simulink model "P3"  (R2017b)
settings: Solver=VariableStepAuto  StartTime=0.0  StopTime=10.0  RelTol=1e-3
values from neighbouring files (symbols this model uses):
  a = [0 1;-1 -0.7]    [P2a.m]    (also in P2b.m; P2c.m)
  b = [0;1]    [P2a.m]    (also in P2b.m; P2c.m)
  c = [1 0;0 0]    [P2a.m]    (also in P2b.m; P2c.m = [1 0)
  P0 = 100*eye(2)    [P2c.m]
  Q = eye(2)    [P2a.m]    (also in P2b.m; P2c.m)
  R = eye(1)    [P2a.m]    (also in P2b.m; P2c.m)
undefined symbols (not defined in the file or in its folder): H_k1, K, L
settings Model: Creator=Soutrik  LastModifiedBy=Soutrik

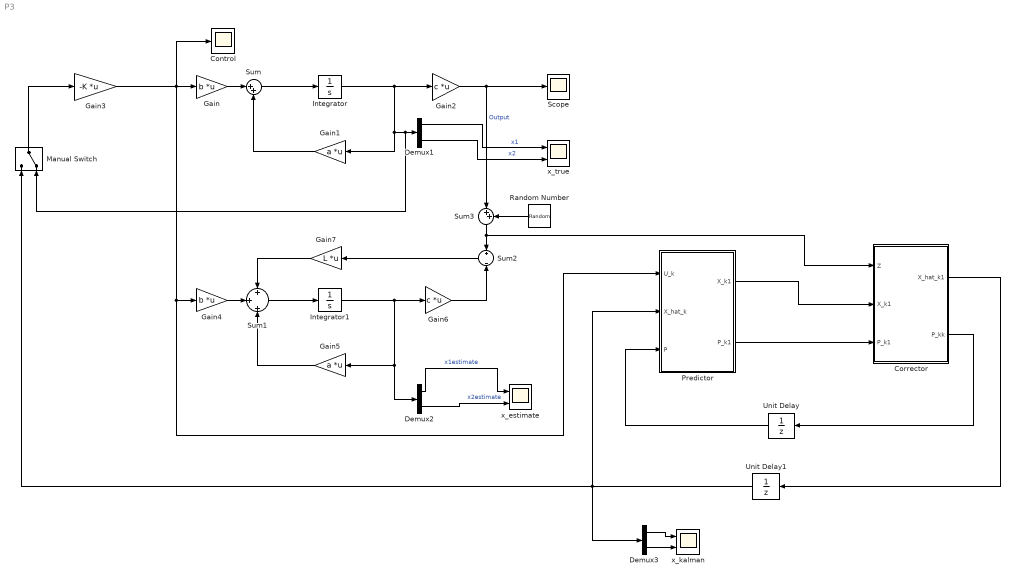
== system P3 ==
  Control : Scope
  Corrector : MATLAB Function  TreatAsAtomicUnit=on
  Demux1 : Demux  Outputs=2
  Demux2 : Demux  Outputs=2
  Demux3 : Demux  Outputs=2
  Gain : Gain  Gain=b  Multiplication=Matrix(K*u)
  Gain1 : Gain  Gain=a  Multiplication=Matrix(K*u)
  Gain2 : Gain  Gain=c  Multiplication=Matrix(K*u)
  Gain3 : Gain  Gain=-K  Multiplication=Matrix(K*u)
  Gain4 : Gain  Gain=b  Multiplication=Matrix(K*u)
  Gain5 : Gain  Gain=a  Multiplication=Matrix(K*u)
  Gain6 : Gain  Gain=c  Multiplication=Matrix(K*u)
  Gain7 : Gain  Gain=L  Multiplication=Matrix(K*u)
  Integrator : Integrator  InitialCondition=[1 0]
  Integrator1 : Integrator  InitialCondition=[1 0]
  Manual Switch : ManualSwitch  CurrentSetting=0
  Predictor : MATLAB Function  TreatAsAtomicUnit=on
  Random Number : RandomNumber  Variance=[0.1,0.1]  Seed=[1 2]  SampleTime=0.01
  Scope : Scope
  Sum : Sum  Inputs=|++
  Sum1 : Sum  Inputs=+|+|+
  Sum2 : Sum  Inputs=+||-
  Sum3 : Sum  Inputs=|++
  Unit Delay : UnitDelay  InitialCondition=P0  SampleTime=-1
  Unit Delay1 : UnitDelay  InitialCondition=[1 0]  SampleTime=-1
  x_estimate : Scope  NumInputPorts=2
  x_kalman : Scope  NumInputPorts=2
  x_true : Scope  NumInputPorts=2
  wires:
  Manual Switch/1 -> Gain3/1
  Corrector/1(X_hat_k1) -> Unit Delay1/1
  Predictor/2(P_k1) -> Corrector/3(P_k1)
  Demux3/1 -> x_kalman/1
  Sum2/1 -> Gain7/1
  Demux2/1 -> x_estimate/1  "x1estimate"
  Unit Delay/1 -> Predictor/3(P)
  Integrator1/1 -> Gain5/1, Demux2/1, Gain6/1
  Unit Delay1/1 -> Manual Switch/1, Demux3/1, Predictor/2(X_hat_k)
  Gain7/1 -> Sum1/1
  Corrector/2(P_kk) -> Unit Delay/1
  Gain3/1 -> Predictor/1(U_k), Gain4/1, Gain/1, Control/1
  Gain5/1 -> Sum1/3
  Demux2/2 -> x_estimate/2  "x2estimate"
  Gain6/1 -> Sum2/2
  Integrator/1 -> Gain1/1, Manual Switch/2, Demux1/1, Gain2/1
  Sum3/1 -> Corrector/1(Z), Sum2/1
  Demux1/1 -> x_true/1  "x1"
  Demux1/2 -> x_true/2  "x2"
  Demux3/2 -> x_kalman/2
  Sum/1 -> Integrator/1
  Gain2/1 -> Scope/1, Sum3/1  "Output"
  Gain4/1 -> Sum1/2
  Random Number/1 -> Sum3/2
  Gain1/1 -> Sum/2
  Predictor/1(X_k1) -> Corrector/2(X_k1)
  Sum1/1 -> Integrator1/1
  Gain/1 -> Sum/1

== matlab function P3/Corrector ==
  data: Z input size=2; X_k1 input size=2; X_hat_k1 output size=2; P_k1 input size=[2 2]; P_kk output size=[2 2]; H_k1 parameter size=[2 2]; R parameter
function [X_hat_k1,P_kk]= fcn(Z,X_k1,P_k1,H_k1, R)
R_k1 = R./0.01;

K_k1 = P_k1 * H_k1' * inv(H_k1 * P_k1 * H_k1' + R_k1);

P_kk = (eye(2) - K_k1 * H_k1) * P_k1 * (eye(2) - K_k1 * H_k1)' + K_k1 * R_k1 * K_k1';

X_hat_k1 = X_k1 + K_k1 * (Z - H_k1 * X_k1);

== matlab function P3/Predictor ==
  data: U_k input size=1; X_k1 output size=2; X_hat_k input size=2; P_k1 output size=[2 2]; a parameter; b parameter; Q parameter; P input size=[2 2]
function [X_k1,P_k1]= fcn(U_k,X_hat_k,a, b,Q, P)

Ak = expm(a * 0.01);
Bk = inv(a) * (Ak - eye(2)) * b;
F = [-a Q;
     zeros(2) a';];
F = F*0.01;
G = expm(F);
Qk = G(3:4,3:4)'*G(1:2,3:4);

X_k1 = Ak * X_hat_k + Bk * U_k;
P_k1 = Ak * P * Ak' + Qk;
